simulink subsystem "power_window_system_impact"  (R2021a)
settings: Solver=VariableStepAuto  StartTime=0.0  StopTime=10.0  RelTol=1e-3
undefined symbols (not defined in the file): B, Ke_phi, Ra, tau_a1, tau_m, TL
settings Model: Creator=achu  LastModifiedBy=Sai229

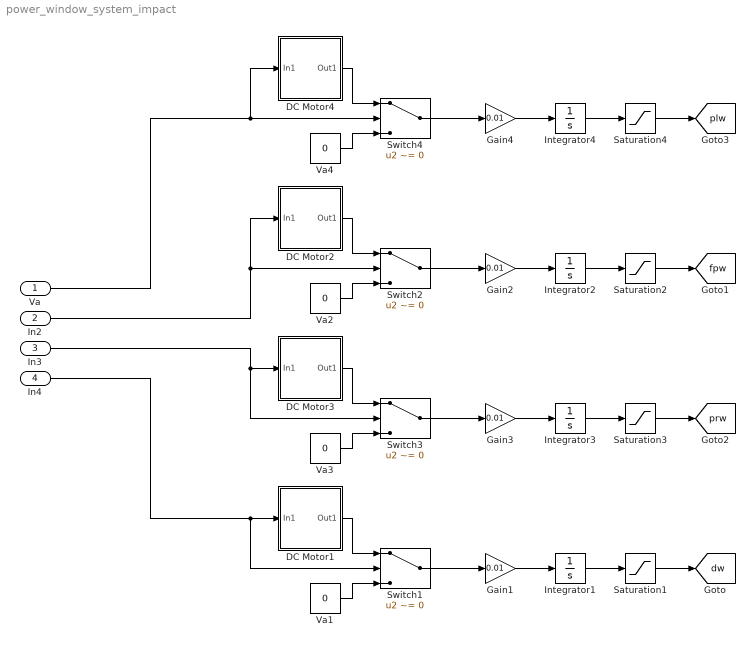
== system power_window_system_impact ==
  Va : Inport
  In2 : Inport  Port=2
  In3 : Inport  Port=3
  In4 : Inport  Port=4
  DC Motor1 : Subsystem
  DC Motor2 : Subsystem
  DC Motor3 : Subsystem
  DC Motor4 : Subsystem
  Gain{1..4} (4 alike) : Gain  Gain=0.01
  Integrator{1..4} (4 alike) : Integrator
  Saturation{1..4} (4 alike) : Saturate  UpperLimit=10  LowerLimit=0
  Switch{1..4} (4 alike) : Switch  Criteria=u2 ~= 0
  Va{1..4} (4 alike) : Constant  Value=0
  tag scope: dw=global, fpw=global, plw=global, prw=global
  wires:
  DC Motor1/1(Out1) -> Switch1/1
  Saturation1/1 -> [dw]
  Saturation4/1 -> [plw]
  Va1/1 -> Switch1/3
  Gain1/1 -> Integrator1/1
  Integrator3/1 -> Saturation3/1
  Va2/1 -> Switch2/3
  Va4/1 -> Switch4/3
  Integrator4/1 -> Saturation4/1
  Switch3/1 -> Gain3/1
  In4/1 -> DC Motor1/1(In1), Switch1/2
  Integrator2/1 -> Saturation2/1
  Gain4/1 -> Integrator4/1
  DC Motor4/1(Out1) -> Switch4/1
  Saturation2/1 -> [fpw]
  Switch4/1 -> Gain4/1
  Integrator1/1 -> Saturation1/1
  In2/1 -> Switch2/2, DC Motor2/1(In1)
  Va3/1 -> Switch3/3
  In3/1 -> DC Motor3/1(In1), Switch3/2
  DC Motor3/1(Out1) -> Switch3/1
  Switch1/1 -> Gain1/1
  Switch2/1 -> Gain2/1
  Gain3/1 -> Integrator3/1
  Saturation3/1 -> [prw]
  Gain2/1 -> Integrator2/1
  DC Motor2/1(Out1) -> Switch2/1
  Va/1 -> Switch4/2, DC Motor4/1(In1)

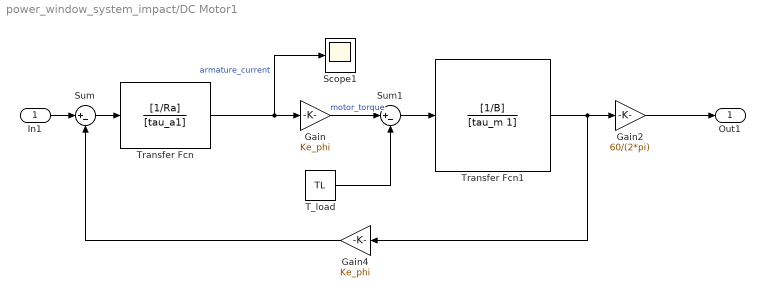
== system power_window_system_impact/DC Motor1 ==
  In1 : Inport
  Gain : Gain  Gain=Ke_phi
  Gain2 : Gain  Gain=60/(2*pi)
  Gain4 : Gain  Gain=Ke_phi
  Scope1 : Scope
  Sum : Sum  Inputs=|+-
  Sum1 : Sum  Inputs=|+-
  T_load : Constant  Value=TL
  Transfer Fcn : TransferFcn  Numerator=[1/Ra]  Denominator=[tau_a1]
  Transfer Fcn1 : TransferFcn  Numerator=[1/B]  Denominator=[tau_m 1]
  Out1 : Outport
  wires:
  Gain/1 -> Sum1/1  "motor_torque"
  Transfer Fcn1/1 -> Gain2/1, Gain4/1
  T_load/1 -> Sum1/2
  Transfer Fcn/1 -> Gain/1, Scope1/1  "armature_current"
  Gain4/1 -> Sum/2
  Gain2/1 -> Out1/1
  Sum/1 -> Transfer Fcn/1
  Sum1/1 -> Transfer Fcn1/1
  In1/1 -> Sum/1

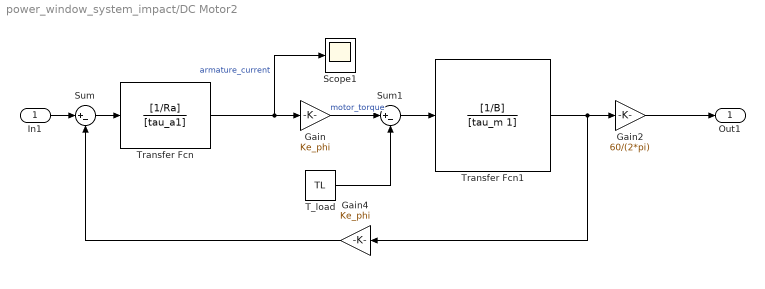
== system power_window_system_impact/DC Motor2 ==
  In1 : Inport
  Gain : Gain  Gain=Ke_phi
  Gain2 : Gain  Gain=60/(2*pi)
  Gain4 : Gain  Gain=Ke_phi
  Scope1 : Scope
  Sum : Sum  Inputs=|+-
  Sum1 : Sum  Inputs=|+-
  T_load : Constant  Value=TL
  Transfer Fcn : TransferFcn  Numerator=[1/Ra]  Denominator=[tau_a1]
  Transfer Fcn1 : TransferFcn  Numerator=[1/B]  Denominator=[tau_m 1]
  Out1 : Outport
  wires:
  Gain/1 -> Sum1/1  "motor_torque"
  Transfer Fcn1/1 -> Gain2/1, Gain4/1
  T_load/1 -> Sum1/2
  Transfer Fcn/1 -> Gain/1, Scope1/1  "armature_current"
  Gain4/1 -> Sum/2
  Gain2/1 -> Out1/1
  Sum/1 -> Transfer Fcn/1
  Sum1/1 -> Transfer Fcn1/1
  In1/1 -> Sum/1

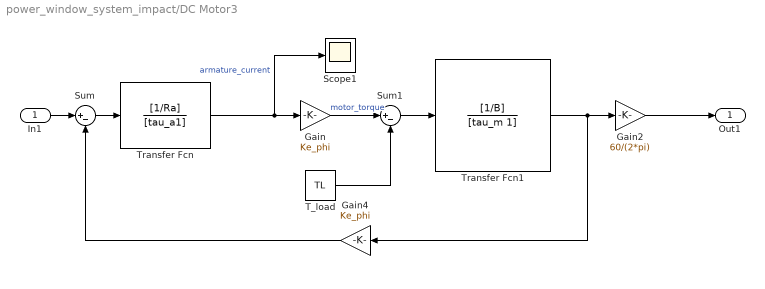
== system power_window_system_impact/DC Motor3 ==
  In1 : Inport
  Gain : Gain  Gain=Ke_phi
  Gain2 : Gain  Gain=60/(2*pi)
  Gain4 : Gain  Gain=Ke_phi
  Scope1 : Scope
  Sum : Sum  Inputs=|+-
  Sum1 : Sum  Inputs=|+-
  T_load : Constant  Value=TL
  Transfer Fcn : TransferFcn  Numerator=[1/Ra]  Denominator=[tau_a1]
  Transfer Fcn1 : TransferFcn  Numerator=[1/B]  Denominator=[tau_m 1]
  Out1 : Outport
  wires:
  Gain/1 -> Sum1/1  "motor_torque"
  Transfer Fcn1/1 -> Gain2/1, Gain4/1
  T_load/1 -> Sum1/2
  Transfer Fcn/1 -> Gain/1, Scope1/1  "armature_current"
  Gain4/1 -> Sum/2
  Gain2/1 -> Out1/1
  Sum/1 -> Transfer Fcn/1
  Sum1/1 -> Transfer Fcn1/1
  In1/1 -> Sum/1

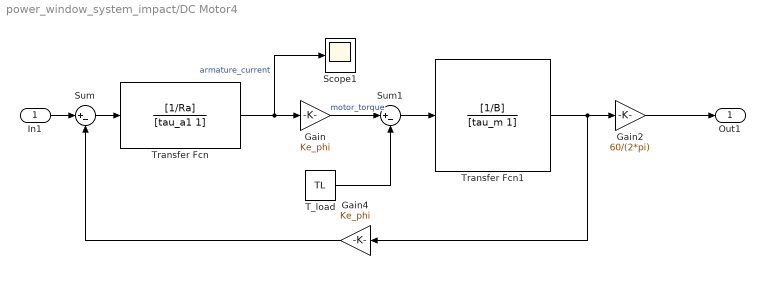
== system power_window_system_impact/DC Motor4 ==
  In1 : Inport
  Gain : Gain  Gain=Ke_phi
  Gain2 : Gain  Gain=60/(2*pi)
  Gain4 : Gain  Gain=Ke_phi
  Scope1 : Scope
  Sum : Sum  Inputs=|+-
  Sum1 : Sum  Inputs=|+-
  T_load : Constant  Value=TL
  Transfer Fcn : TransferFcn  Numerator=[1/Ra]  Denominator=[tau_a1 1]
  Transfer Fcn1 : TransferFcn  Numerator=[1/B]  Denominator=[tau_m 1]
  Out1 : Outport
  wires:
  Gain/1 -> Sum1/1  "motor_torque"
  Transfer Fcn1/1 -> Gain2/1, Gain4/1
  T_load/1 -> Sum1/2
  Transfer Fcn/1 -> Gain/1, Scope1/1  "armature_current"
  Gain4/1 -> Sum/2
  Gain2/1 -> Out1/1
  Sum/1 -> Transfer Fcn/1
  Sum1/1 -> Transfer Fcn1/1
  In1/1 -> Sum/1
